simulink library "SEA_library_controllers_experimental"  (Simulink 8.6)
settings: Solver=VariableStepAuto  StartTime=0.0  StopTime=10.0  RelTol=1e-3
undefined symbols (not defined in the file or in its folder): Ar, Br, Cr, DiscIntNeverNeededParam, K_lqr, V
undefined symbols (not defined in the file): My_joint
libraries: SEA_library_observers x2, cstblocks x1
settings Model: Creator=wesley  LastModifiedBy=wesley

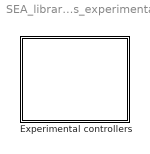
== system SEA_library_controllers_experimental ==
  Experimental controllers : Subsystem

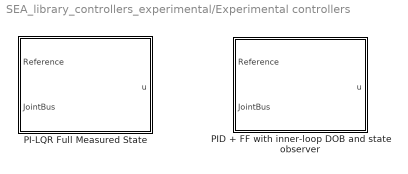
== system SEA_library_controllers_experimental/Experimental controllers ==
  PI-LQR Full Measured State : Subsystem  mask{jointObj=My_joint, Q=diag([0 1 0 0 1e-6]), R=1e-9}
      mask prompts: jointObj "Joint Object (fixed output model)"; Q "State weighing matrix Q"; R "Input weighing matrix R"
      mask init:
      | % Get linear dynamics matrices
      | [A, B, C, I, D, K] = jointObj.getDynamicsMatrices();
      | 
      | [ K_lqr, V, Ar, Br, Cr] = mask_PI_LQR_Full_Measured_State( jointObj, Q, R )
  PID + FF with inner-loop DOB and state observer : Subsystem  mask{jointObj=My_joint, Kp=0.14, Ki=0, Kd=0.10, N=2*pi*200, measIdx=[2], f_c=100, Q=diag([0 1000 0 0]), R=5e-6, place_gain=4, doPlot=off}
      mask prompts: jointObj "Joint Object"; Kp "Proportional gain Kp"; Ki "Integral gain Ki"; Kd "Derivative gain Kd"; N "Filter coefficient N"; measIdx "Measurement index"; f_c "DOB cut-off frequency [Hz]"; Q "State weighing matrix Q"; R "Input weighing matrix R"; place_gain "Pole placement gain"; doPlot "Do plot"
      mask init:
      | % Get linear dynamics matrices
      | [A, B, C, I, D, K] = jointObj.getDynamicsMatrices();
      mask DialogControl DOB_container Prompt: DOB
      mask DialogControl Observer_container Prompt: State observer

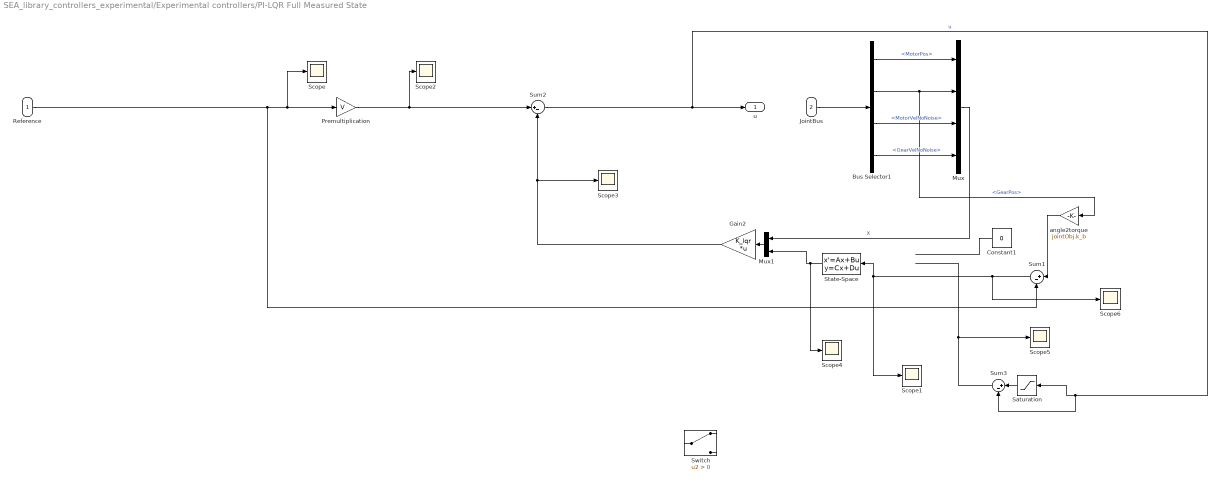
== system SEA_library_controllers_experimental/Experimental controllers/PI-LQR Full Measured State ==
  Reference : Inport
  JointBus : Inport  Port=2
  Bus Selector1 : BusSelector  OutputSignals=MotorPos,GearPos,MotorVelNoNoise,GearVelNoNoise
  Constant1 : Constant  Value=0
  Gain2 : Gain  Gain=K_lqr  Multiplication=Matrix(K*u)
  Mux : Mux
  Mux1 : Mux  Inputs=2
  Premultiplication : Gain  Gain=V
  Saturation : Saturate  UpperLimit=40  LowerLimit=-40
  Scope{,1..6} (7 alike) : Scope
  State-Space : StateSpace  A=Ar  B=Br  C=Cr  D=0  X0=0
  Sum1 : Sum  Inputs=|+-
  Sum2 : Sum  Inputs=|+-
  Sum3 : Sum  Inputs=|+-
  Switch : Switch  Criteria=u2 > Threshold
  angle2torque : Gain  Gain=jointObj.k_b
  u : Outport
  wires:
  Sum1/1 -> Scope6/1, Scope1/1, State-Space/1
  Sum3/1 -> Scope5/1
  Saturation/1 -> Sum3/1
  Constant1/1 -> ?
  angle2torque/1 -> Sum1/1
  State-Space/1 -> Mux1/2, Scope4/1
  Mux1/1 -> Gain2/1
  Gain2/1 -> Sum2/2, Scope3/1
  Premultiplication/1 -> Scope2/1, Sum2/1
  JointBus/1 -> Bus Selector1/1
  Mux/1 -> Mux1/1  "X"
  Bus Selector1/1 -> Mux/1  "<MotorPos>"
  Bus Selector1/2 -> Mux/2, angle2torque/1  "<GearPos>"
  Bus Selector1/4 -> Mux/4  "<GearVelNoNoise>"
  Bus Selector1/3 -> Mux/3  "<MotorVelNoNoise>"
  Sum2/1 -> u/1, Saturation/1, Sum3/2  "u"
  Reference/1 -> Scope/1, Premultiplication/1, Sum1/2

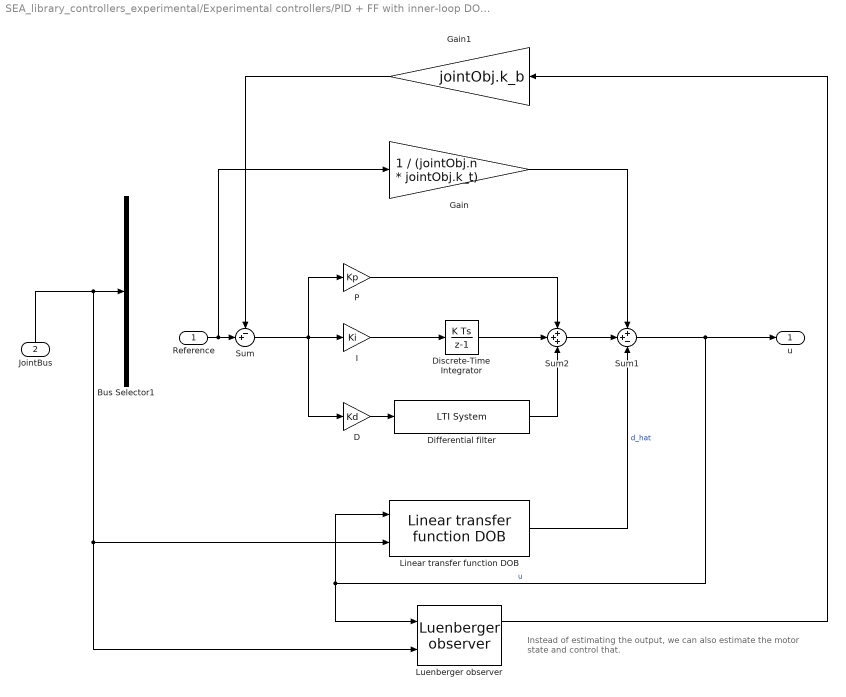
== system SEA_library_controllers_experimental/Experimental controllers/PID + FF with inner-loop DOB and state observer ==
  note: Instead of estimating the output, we can also estimate the motor
      | state and control that.
  Reference : Inport
  JointBus : Inport  Port=2
  Bus Selector1 : BusSelector  OutputSignals=GearPos
  D : Gain  Gain=Kd
  Differential filter : cstblocks/LTI System  sys=c2d(tf([N 0], [1, N]), jointObj.Ts, 'tustin')  IC=[]
  Discrete-Time Integrator : DiscreteIntegrator  SampleTime=jointObj.Ts  ICPrevOutput=DiscIntNeverNeededParam  ICPrevScaledInput=DiscIntNeverNeededParam
  Gain : Gain  Gain=1 / (jointObj.n * jointObj.k_t)
  Gain1 : Gain  Gain=jointObj.k_b
  I : Gain  Gain=Ki
  Linear transfer function DOB : SEA_library_observers/Observers/Linear transfer function DOB  loadData=off  modelFname=DOB_results.mat  jointObj=jointObj  f_c=f_c  measIdx=measIdx  doPlot=off
  Luenberger observer : SEA_library_observers/Observers/Luenberger observer  jointObj=jointObj  outputs_measured=measIdx  Q=Q  R=R  place_gain=place_gain
  P : Gain  Gain=Kp
  Sum : Sum  Inputs=-+|
  Sum1 : Sum  Inputs=++-
  Sum2 : Sum  Inputs=+++
  u : Outport
  wires:
  Sum/1 -> P/1, I/1, D/1
  Sum2/1 -> Sum1/2
  Differential filter/1 -> Sum2/3
  P/1 -> Sum2/1
  Discrete-Time Integrator/1 -> Sum2/2
  I/1 -> Discrete-Time Integrator/1
  D/1 -> Differential filter/1
  Luenberger observer/1 -> Gain1/1
  Linear transfer function DOB/1 -> Sum1/3  "d_hat"
  Reference/1 -> Gain/1, Sum/2
  Gain/1 -> Sum1/1
  JointBus/1 -> Bus Selector1/1, Linear transfer function DOB/2, Luenberger observer/2
  Sum1/1 -> u/1, Luenberger observer/1, Linear transfer function DOB/1  "u"
  Gain1/1 -> Sum/1
